simulink model "HEV_BTP_basic_Perfect_highway_final_25_11_19"  (R2019a)
settings: Solver=VariableStepAuto  StartTime=0  StopTime=198  RelTol=1e-3
undefined symbols (not defined in the file): f_co, f_co2, f_hc, f_nox, f_tbrake_n_bpt, f_tbrake_t_bpt, sigbuilder_block
libraries: fl_lib x100, nesl_utility x32, ee_lib x26, sdl_lib x17, simulink x5
(part 1 of 2)
settings Model: Creator=hp  LastModifiedBy=hp
settings SolverCC: ZeroCrossAlgorithm=Adaptive
settings DataIOCC: ExternalInput=[PedalTime,FrontBrakePedal,RearBrakePedal]  LoadExternalInput=on
settings DebuggingCC: IgnoredZcDiagnostic=none

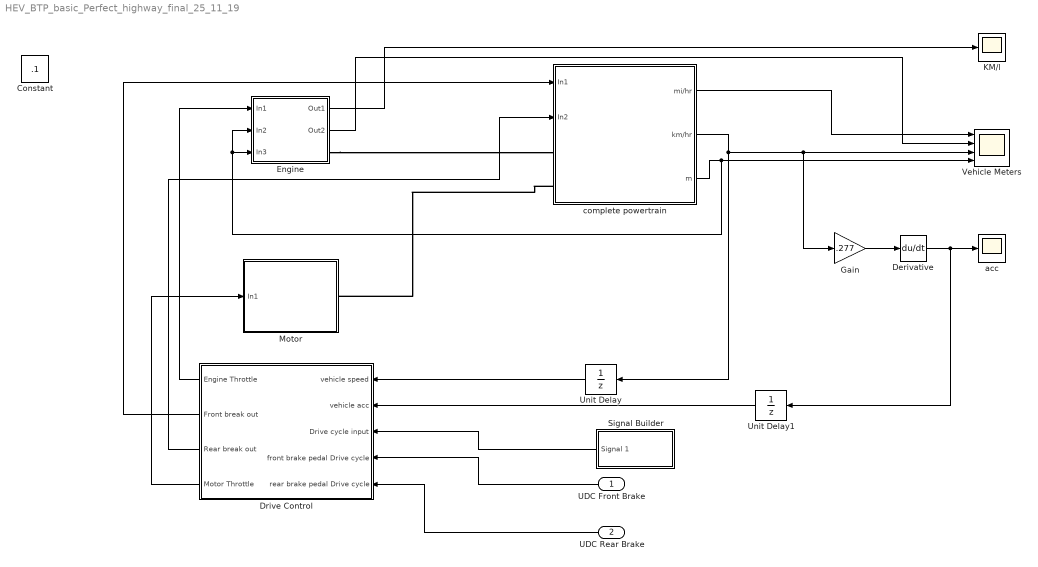
== system HEV_BTP_basic_Perfect_highway_final_25_11_19 ==
  UDC Front Brake : Inport
  UDC Rear Brake : Inport  Port=2
  Constant : Constant  Value=.1
  Derivative : Derivative
  Drive Control : Subsystem
  Engine : Subsystem
  Gain : Gain  Gain=.277
  KM/l : Scope
  Motor : Subsystem
  Signal Builder : Subsystem  Tag=STV Subsys  LoadFcn=sigbuilder_block('load');  StartFcn=sigbuilder_block('start');  StopFcn=sigbuilder_block('stop');  ClipboardFcn=sigbuilder_block('clipboard');  mask(Sigbuilder block){tuvar=[0:10]}
      mask help: Simulink:masks:SigbuilderBlock_MD
      mask init:
      | if ~strcmp(get_param(bdroot(gcbh),'SimulationStatus'),'stopped') tuvar = sigbuilder_block('maskInit'); end
      settings: CopyFcn=sigbuilder_block('copy');  DeleteFcn=sigbuilder_block('delete');  ModelCloseFcn=sigbuilder_block('modelClose');  PreSaveFcn=sigbuilder_block('preSave');  PauseFcn=sigbuilder_block('pause');  ContinueFcn=sigbuilder_block('continue');  NameChangeFcn=sigbuilder_block('namechange');  OpenFcn=sigbuilder_block('open',[6 30 1012.5 447.75 ]);  CloseFcn=sigbuilder_block('close');
      mask Display: plot(0, 0, 100, 100,[2, 2, 32, 32, 2], [68, 8, 8, 68, 68],[32, 2], [38, 38], [32, 19, 2],[53, 60, 44], [32, 17, 17, 2],[16, 16, 31, 31]);txt = getActiveGroup(gcbh);text(2, 100, txt,'verticalAlignment', 'top');
  Unit Delay : UnitDelay  SampleTime=-1  HasFrameUpgradeWarning=on
  Unit Delay1 : UnitDelay  SampleTime=-1  HasFrameUpgradeWarning=on
  "Vehicle Meters " : Scope  NumInputPorts=4
  acc : Scope
  complete powertrain : Subsystem
  wires:
  complete powertrain/2(km/hr) -> Unit Delay/1, Gain/1, "Vehicle Meters "/3
  complete powertrain/1(mi/hr) -> "Vehicle Meters "/1
  complete powertrain/3(m) -> Engine/2(In2), Engine/3(In3), "Vehicle Meters "/4
  Engine/1(Out1) -> KM/l/1
  Engine/2(Out2) -> "Vehicle Meters "/2
  Derivative/1 -> Unit Delay1/1, acc/1
  Gain/1 -> Derivative/1
  Drive Control/4(Motor Throttle) -> Motor/1(In1)
  Drive Control/1(Engine Throttle) -> Engine/1(In1)
  UDC Front Brake/1 -> Drive Control/4(front brake pedal Drive cycle)
  UDC Rear Brake/1 -> Drive Control/5(rear brake pedal Drive cycle)
  Drive Control/2(Front break out) -> complete powertrain/1(In1)
  Drive Control/3(Rear break out) -> complete powertrain/2(In2)
  Unit Delay/1 -> Drive Control/1(vehicle speed)
  Unit Delay1/1 -> Drive Control/2(vehicle acc)
  Signal Builder/1(Signal 1) -> Drive Control/3(Drive cycle input)
  connections:
  Engine/RConn1 -- complete powertrain/LConn1
  complete powertrain/LConn2 -- Motor/RConn1

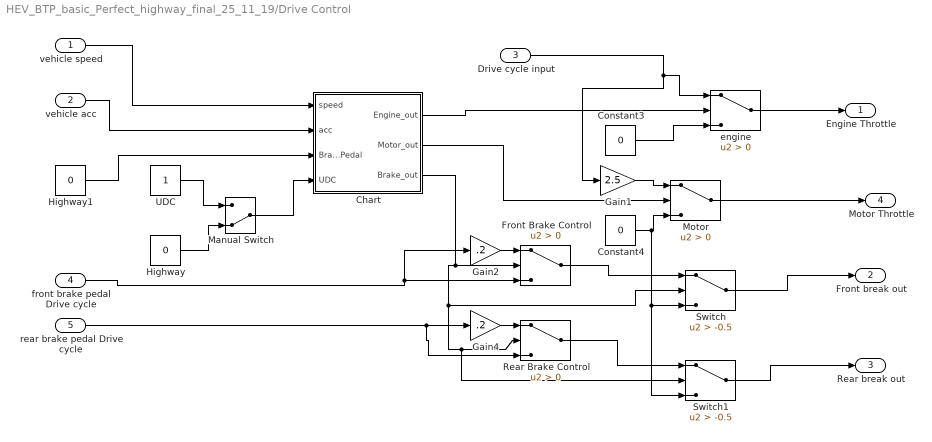
== system HEV_BTP_basic_Perfect_highway_final_25_11_19/Drive Control ==
  vehicle speed : Inport
  vehicle acc : Inport  Port=2
  Drive cycle input : Inport  Port=3
  front brake pedal Drive cycle : Inport  Port=4
  rear brake pedal Drive cycle : Inport  Port=5
  Chart : Stateflow chart  BlockKeywords=__PRM__SERIALIZED__DATA__:Stateflow Chart,Stateflow Diagram  TreatAsAtomicUnit=on
  Constant3 : Constant  Value=0
  Constant4 : Constant  Value=0
  Front Brake Control : Switch  Criteria=u2 > Threshold
  Gain1 : Gain  Gain=2.5
  Gain2 : Gain  Gain=.2
  Gain4 : Gain  Gain=.2
  Highway : Constant  Value=0
  Highway1 : Constant  Value=0
  Manual Switch : ManualSwitch  CurrentSetting=0
  Motor : Switch  Criteria=u2 > Threshold
  Rear Brake Control : Switch  Criteria=u2 > Threshold
  Switch : Switch  Criteria=u2 > Threshold  Threshold=-0.5
  Switch1 : Switch  Criteria=u2 > Threshold  Threshold=-0.5
  UDC : Constant
  engine : Switch  Criteria=u2 > Threshold
  Engine Throttle : Outport
  Front break out : Outport  Port=2
  Rear break out : Outport  Port=3
  Motor Throttle : Outport  Port=4
  wires:
  rear brake pedal Drive cycle/1 -> Rear Brake Control/3, Gain4/1
  Gain4/1 -> Rear Brake Control/1
  front brake pedal Drive cycle/1 -> Gain2/1, Front Brake Control/3
  Gain1/1 -> Motor/1
  Gain2/1 -> Front Brake Control/1
  UDC/1 -> Manual Switch/1
  Chart/2(Motor_out) -> Motor/2
  Chart/3(Brake_out) -> Front Brake Control/2, Switch/2, Switch1/2, Rear Brake Control/2
  Constant4/1 -> Switch1/3, Switch/3, Motor/3
  Highway/1 -> Manual Switch/2
  vehicle speed/1 -> Chart/1(speed)
  Drive cycle input/1 -> Gain1/1, engine/1
  engine/1 -> Engine Throttle/1
  Chart/1(Engine_out) -> engine/2
  Manual Switch/1 -> Chart/4(UDC)
  Constant3/1 -> engine/3
  Motor/1 -> Motor Throttle/1
  vehicle acc/1 -> Chart/2(acc)
  Front Brake Control/1 -> Switch/1
  Switch/1 -> Front break out/1
  Switch1/1 -> Rear break out/1
  Rear Brake Control/1 -> Switch1/1
  Highway1/1 -> Chart/3(Brake_Pedal)

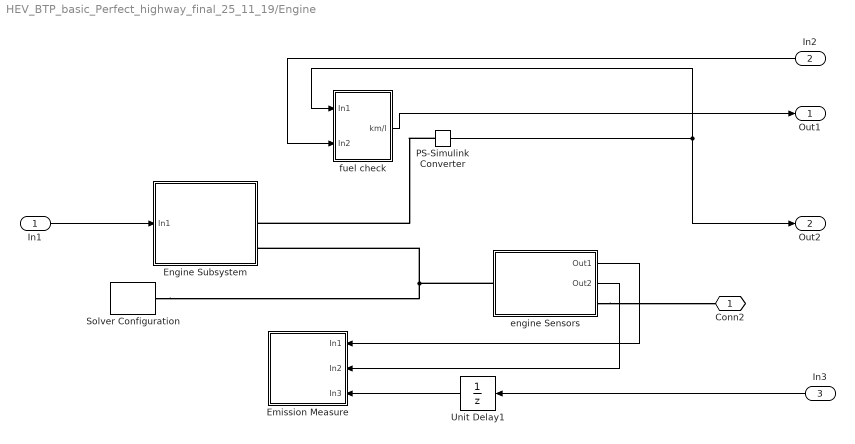
== system HEV_BTP_basic_Perfect_highway_final_25_11_19/Engine ==
  In1 : Inport
  In2 : Inport  Port=2
  In3 : Inport  Port=3
  Emission Measure : Subsystem
  Engine Subsystem : Subsystem
  PS-Simulink Converter : nesl_utility/PS-Simulink Converter  PhysicalDomain=network_engine_domain  SubClassName=ps_output  LeftPortType=input  RightPortType=output  PseudoPeriodic=off  Frequencies=[]  Unit=g/s  AffineConversion=off
  Solver Configuration : nesl_utility/Solver Configuration  PhysicalDomain=network_engine_domain  SubClassName=solver  LeftPortType=input  RightPortType=generic  Tones=[]  Harmonics=[]  SimulateNoise=off  Profile=off  UseLocalSampling=off  EnableSwitchedLinearOptims=on  FrequencyDomain=off  UseCCode=off  RelTol=0.001  AbsTol=1e-06  MinStep=1e-09  ToWorkspace=off  RevertToSquareIcSolve=off  NumHomotopyIterations=100  PhasorMode=off  PhasorModeNumHarmonics=1  DoDC=off  ResidualTolerance=1e-09  UseLocalSolver=off  LocalSolverChoice=NE_BACKWARD_EULER_ADVANCER  LocalSolverSampleTime=0.001  DoFixedCost=off  MaxNonlinIter=3  MaxModeIter=2  LinearAlgebra=auto  EquationFormulation=NE_TIME_EF  DelaysMemoryBudget=1024  AutomaticFiltering=on  FilteringTimeConstant=0.001  PartitionStorageMethod=AS_NEEDED  PartitionMemoryBudget=1024  PartitionMethod=ROBUST
  Unit Delay1 : UnitDelay  SampleTime=-1  HasFrameUpgradeWarning=on
  engine Sensors : Subsystem
  "fuel check " : Subsystem
  Conn2 : PMIOPort  Side=Right
  Out1 : Outport
  Out2 : Outport  Port=2
  wires:
  engine Sensors/1(Out1) -> Emission Measure/1(In1)
  Unit Delay1/1 -> Emission Measure/3(In3)
  "fuel check "/1(km/l) -> Out1/1
  engine Sensors/2(Out2) -> Emission Measure/2(In2)
  PS-Simulink Converter/1 -> Out2/1, "fuel check "/1(In1)
  In2/1 -> "fuel check "/2(In2)
  In3/1 -> Unit Delay1/1
  In1/1 -> Engine Subsystem/1(In1)
  connections:
  Solver Configuration/RConn1 -- engine Sensors/LConn1 -- Engine Subsystem/RConn3
  PS-Simulink Converter/LConn1 -- Engine Subsystem/RConn2
  engine Sensors/RConn1 -- Conn2/RConn1

== system HEV_BTP_basic_Perfect_highway_final_25_11_19/Motor ==
  In1 : Inport
  Battery Subsystem : Subsystem
  DC Motor : Subsystem
  Motor Sensors : Subsystem
  Conn1 : PMIOPort  Side=Right
  wires:
  In1/1 -> Battery Subsystem/1(Pedal Input)
  connections:
  Motor Sensors/LConn1 -- DC Motor/RConn1
  DC Motor/LConn1 -- Battery Subsystem/RConn1
  DC Motor/LConn2 -- Battery Subsystem/RConn2
  Motor Sensors/RConn1 -- Conn1/RConn1

== system HEV_BTP_basic_Perfect_highway_final_25_11_19/Signal Builder ==
  Demux : Demux  Tag=STV Demux  Outputs=1
  FromWs : FromWorkspace  Tag=STV FromWs  VariableName=tuvar  SampleTime=0
      SigBuilderData=|
      | common.afterFinalStr = 'Extrapolate'
      | common.sampleTime = 0
      | dataSet.timeRange = [0 200]
      | dataSet.name = 'Group 1'
      | sbobj.Groups.Name = 'Group 1'
      | sbobj.Groups.Signals.Name = 'Signal 1'
      | sbobj.Groups.Signals.XData = [0 3.33333333333 3.33333333333 6.66666666667 6.66666666667 12.6 14.8 16.6666666667 16.6666666667 20 23.3333333333 26.6666666667 30 33.3333333333 33.3333333333 36.6666666667 40 40 43.3333333333 46.6666666667 50 50 53.3333333333 56.6666666667 60 60 63.3333333333 63.3333333333 66.6666666667 66.6666666667 70 73.3333333333 76.6666666667 80 80 83.3333333333 86.6666666667 86.6666666667 90 90 93.3333333333 96.6666666667 96.6666666667 100 100 103.333333333 106.666666667 110 110 113.333333333 116.666666667 116.666666667 120 120 123.333333333 123.333333333 126.666666667 130 130 133.333333333 136.666666667 140 143.333333333 143.333333333 146.666666667 150 153.333333333 153.333333333 156.666666667 156.666666667 160 163.333333333 166.666666667 171 171 173.333333333 173.333333333 176.666666667 180 180 183.333333333 183.333333333 186.666666667 186.666666667 190 190 193.333333333 193.333333333 196.666666667 200]
      | sbobj.Groups.Signals.YData = [0.01 0.1 0.11 0.16 0.17 0.17 0.14 0.14 0.13 0.13 0.16 0.16 0.19 0.22 0.23 0.24 0.25 0.24 0.19 0.14 0.14 0.15 0.15 0.15 0.15 0.14 0.17 0.18 0.23 0.24 0.27 0.27 0.27 0.27 0.28 0.28 0.28 0.27 0.27 0.26 0.26 0.26 0.28 0.34 0.35 0.35 0.42 0.42 0.43 0.43 0.39 0.38 0.3 0.29 0.22 0.21 0.13 0.01 0 0 0 0.02 0.02 0.03 0.1 0.13 0.17 0.18 0.21 0.22 0.22 0.28 0.35 0.4 0.41 0.48 0.49 0.53 0.57 0.59 0.59 0.6 0.6 0.59 0.59 0.6 0.6 0.61 0.61 0.61]
      | sbobj.Groups.TimeRange = [0 200]
  Signal 1 : Outport  Tag=STV Outport
  wires:
  FromWs/1 -> Demux/1
  Demux/1 -> Signal 1/1

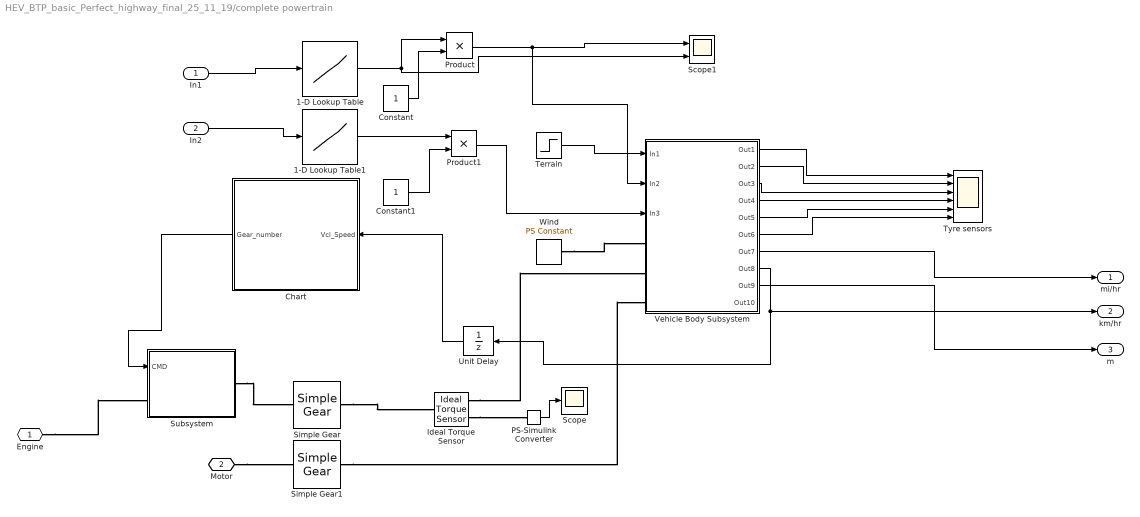
== system HEV_BTP_basic_Perfect_highway_final_25_11_19/complete powertrain ==
  In1 : Inport
  In2 : Inport  Port=2
  1-D Lookup Table : Lookup_n-D  NumberOfTableDimensions=1  BreakpointsForDimension1=0:0.01:1  Table=0:10:1000  InternalRulePriority=Speed  RndMeth=Simplest  InputSameDT=on
  1-D Lookup Table1 : Lookup_n-D  NumberOfTableDimensions=1  BreakpointsForDimension1=0:0.01:1  Table=0:10:1000  InternalRulePriority=Speed  RndMeth=Simplest  InputSameDT=on
  Chart : Stateflow chart  BlockKeywords=__PRM__SERIALIZED__DATA__:Stateflow Chart,Stateflow Diagram  TreatAsAtomicUnit=on
  Constant : Constant
  Constant1 : Constant
  Ideal Torque Sensor : fl_lib/Mechanical/Mechanical Sensors/Ideal Torque Sensor
  PS-Simulink Converter : nesl_utility/PS-Simulink Converter  PhysicalDomain=network_engine_domain  SubClassName=ps_output  LeftPortType=input  RightPortType=output  PseudoPeriodic=off  Frequencies=[]  Unit=N*m  AffineConversion=off
  Product : Product
  Product1 : Product
  Scope : Scope
  Scope1 : Scope  NumInputPorts=2
  Simple Gear : sdl_lib/Gears/Simple Gear  ratio=6  rotation_direction=1  friction_model=sdl.enum.gear_efficiencies_load.off  T_noload=0.1 N*m  T_nom=5 N*m  efficiency_nom=0.8  efficiency=0.8  mu_visc=[0, 0] N*m/(rad/s)  w_thr=0.01 rad/s  pwr_thr=0.001 W  enable_faults=simscape.enum.onoff.off  efficiency_fault=0.05  external_fault=simscape.enum.onoff.off  temporal_fault=simscape.enum.onoff.off  fault_time=5 s  fault_angles=pi / 12 rad  report_fault=1  temperature_TLU=[280, 300, 320] K  load_TLU=[1, 5, 10] N*m  efficiency_TLU=[.95, .9, .85]  efficiency_TLU2=[.85, .8, .75; .95, .9, .85; .85, .8, .7]  thermal_mass=50 J/K  T_init=300 K
      settings: SourceProductName=Simscape Driveline
  Simple Gear1 : sdl_lib/Gears/Simple Gear  ratio=12  rotation_direction=1  friction_model=sdl.enum.gear_efficiencies_load.off  T_noload=0.1 N*m  T_nom=5 N*m  efficiency_nom=0.8  efficiency=0.8  mu_visc=[0, 0] N*m/(rad/s)  w_thr=0.01 rad/s  pwr_thr=0.001 W  enable_faults=simscape.enum.onoff.off  efficiency_fault=0.05  external_fault=simscape.enum.onoff.off  temporal_fault=simscape.enum.onoff.off  fault_time=5 s  fault_angles=pi / 12 rad  report_fault=1  temperature_TLU=[280, 300, 320] K  load_TLU=[1, 5, 10] N*m  efficiency_TLU=[.95, .9, .85]  efficiency_TLU2=[.85, .8, .75; .95, .9, .85; .85, .8, .7]  thermal_mass=50 J/K  T_init=300 K
      settings: SourceProductName=Simscape Driveline
  Subsystem : Subsystem
  Terrain : Step  Time=700  Before=-0.5*(pi/180)  After=0  SampleTime=0
  Tyre sensors : Scope  NumInputPorts=6
  Unit Delay : UnitDelay  SampleTime=.05  HasFrameUpgradeWarning=on
  Vehicle Body Subsystem : Subsystem
  "Wind " : fl_lib/Physical Signals/Sources/PS Constant  constant=3 m/s
  Engine : PMIOPort  Side=Left
  Motor : PMIOPort  Port=2  Side=Left
  mi/hr : Outport
  km/hr : Outport  Port=2
  m : Outport  Port=3
  wires:
  Terrain/1 -> Vehicle Body Subsystem/1(In1)
  Vehicle Body Subsystem/1(Out1) -> Tyre sensors/1
  Vehicle Body Subsystem/3(Out3) -> Tyre sensors/3
  Vehicle Body Subsystem/6(Out6) -> Tyre sensors/6
  Vehicle Body Subsystem/5(Out5) -> Tyre sensors/5
  Vehicle Body Subsystem/2(Out2) -> Tyre sensors/2
  PS-Simulink Converter/1 -> Scope/1
  Vehicle Body Subsystem/4(Out4) -> Tyre sensors/4
  Chart/1(Gear_number) -> Subsystem/1("CMD ")
  Vehicle Body Subsystem/8(Out8) -> km/hr/1, Unit Delay/1
  Unit Delay/1 -> Chart/1(Vcl_Speed)
  Vehicle Body Subsystem/7(Out7) -> mi/hr/1
  Vehicle Body Subsystem/9(Out9) -> m/1
  In1/1 -> 1-D Lookup Table/1
  In2/1 -> 1-D Lookup Table1/1
  1-D Lookup Table/1 -> Product/1, Scope1/2
  Constant/1 -> Product/2
  Product/1 -> Vehicle Body Subsystem/2(In2), Scope1/1
  1-D Lookup Table1/1 -> Product1/1
  Constant1/1 -> Product1/2
  Product1/1 -> Vehicle Body Subsystem/3(In3)
  connections:
  Ideal Torque Sensor/RConn1 -- Vehicle Body Subsystem/LConn2
  "Wind "/RConn1 -- Vehicle Body Subsystem/LConn1
  Subsystem/RConn1 -- Simple Gear/LConn1
  Ideal Torque Sensor/RConn2 -- PS-Simulink Converter/LConn1
  Engine/RConn1 -- Subsystem/LConn1
  Simple Gear/RConn1 -- Ideal Torque Sensor/LConn1
  Simple Gear1/RConn1 -- Vehicle Body Subsystem/LConn3
  Motor/RConn1 -- Simple Gear1/LConn1

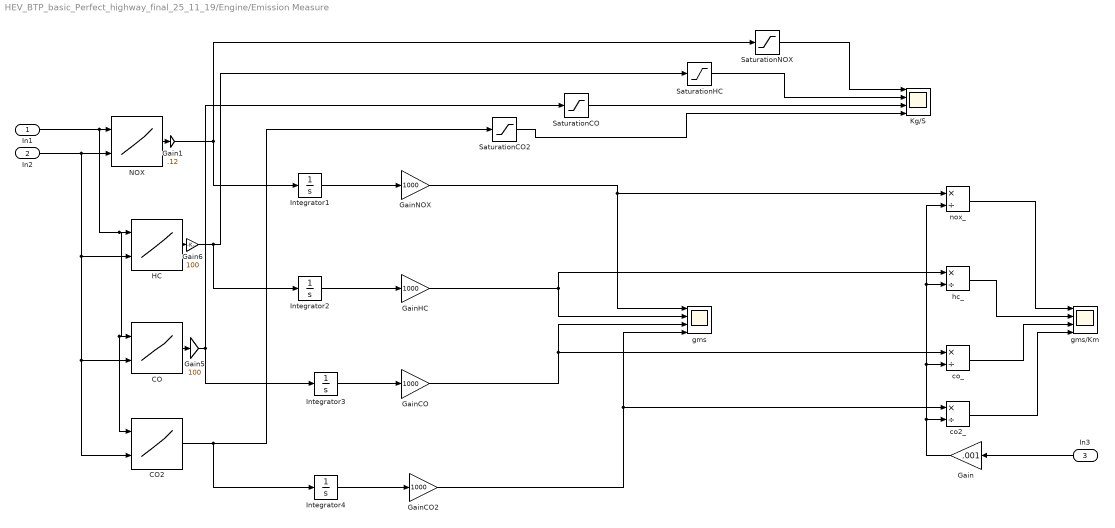
== system HEV_BTP_basic_Perfect_highway_final_25_11_19/Engine/Emission Measure ==
  In1 : Inport
  In2 : Inport  Port=2
  In3 : Inport  Port=3
  CO : Lookup_n-D  BreakpointsForDimension1=f_tbrake_t_bpt  BreakpointsForDimension2=f_tbrake_n_bpt  Table=f_co  InternalRulePriority=Speed  RndMeth=Simplest  InputSameDT=on
  CO2 : Lookup_n-D  BreakpointsForDimension1=f_tbrake_t_bpt  BreakpointsForDimension2=f_tbrake_n_bpt  Table=f_co2  InternalRulePriority=Speed  RndMeth=Simplest  InputSameDT=on
  Gain : Gain  Gain=.001
  Gain1 : Gain  Gain=.12
  Gain5 : Gain  Gain=100
  Gain6 : Gain  Gain=100
  GainCO : Gain  Gain=1000
  GainCO2 : Gain  Gain=1000
  GainHC : Gain  Gain=1000
  GainNOX : Gain  Gain=1000
  HC : Lookup_n-D  BreakpointsForDimension1=f_tbrake_t_bpt  BreakpointsForDimension2=f_tbrake_n_bpt  Table=f_hc  InternalRulePriority=Speed  RndMeth=Simplest  InputSameDT=on
  Integrator{1..4} (4 alike) : Integrator
  Kg/S : Scope  NumInputPorts=4
  NOX : Lookup_n-D  BreakpointsForDimension1=f_tbrake_t_bpt  BreakpointsForDimension2=f_tbrake_n_bpt  Table=f_nox  InternalRulePriority=Speed  RndMeth=Simplest  InputSameDT=on
  SaturationCO : Saturate  UpperLimit=inf  LowerLimit=0  ZeroCross=off
  SaturationCO2 : Saturate  UpperLimit=inf  LowerLimit=0  ZeroCross=off
  SaturationHC : Saturate  UpperLimit=inf  LowerLimit=0  ZeroCross=off
  SaturationNOX : Saturate  UpperLimit=inf  LowerLimit=0  ZeroCross=off
  co2_ : Product  Inputs=*/
  co_ : Product  Inputs=*/
  gms : Scope  NumInputPorts=4
  gms/Km : Scope  NumInputPorts=4
  hc_ : Product  Inputs=*/
  nox_ : Product  Inputs=*/
  wires:
  NOX/1 -> Gain1/1
  In2/1 -> CO2/2, CO/2, HC/2, NOX/2
  In1/1 -> CO2/1, CO/1, HC/1, NOX/1
  HC/1 -> Gain6/1
  CO/1 -> Gain5/1
  CO2/1 -> SaturationCO2/1, Integrator4/1
  SaturationNOX/1 -> Kg/S/1
  SaturationHC/1 -> Kg/S/2
  SaturationCO2/1 -> Kg/S/4
  SaturationCO/1 -> Kg/S/3
  Gain6/1 -> Integrator2/1, SaturationHC/1
  Gain5/1 -> SaturationCO/1, Integrator3/1
  Integrator3/1 -> GainCO/1
  Integrator4/1 -> GainCO2/1
  Integrator2/1 -> GainHC/1
  Integrator1/1 -> GainNOX/1
  GainCO2/1 -> co2_/1, gms/4
  GainHC/1 -> gms/2, hc_/1
  GainNOX/1 -> nox_/1, gms/1
  GainCO/1 -> gms/3, co_/1
  Gain/1 -> nox_/2, hc_/2, co_/2, co2_/2
  nox_/1 -> gms/Km/1
  hc_/1 -> gms/Km/2
  co_/1 -> gms/Km/3
  co2_/1 -> gms/Km/4
  Gain1/1 -> SaturationNOX/1, Integrator1/1
  In3/1 -> Gain/1

== system HEV_BTP_basic_Perfect_highway_final_25_11_19/Engine/Engine Subsystem ==
  In1 : Inport
  Generic Engine : sdl_lib/Engines/Generic Engine  model_parameterization=1  engine_type=1  P_max=51.5 kW  w_P_max=5500 rpm  w_max=6175 rpm  w_min=500 rpm  w_tab=[500, 1000, 2000, 3000, 4000, 5000, 6000, 7000] rpm  trq_tab=[380, 380, 380, 380, 350, 280, 200, 80] N*m  pwr_tab=[20, 40, 78, 120, 145, 148, 125, 60] kW  interp_method=simscape.enum.interpolation.linear  model_inertia=1  inertia=.5 kg*m^2  initial_velocity=875 rpm  model_time_constant=0  time_constant=0.2 s  T0=0  w_thr=100 rpm  idle_speed=0  idle_speed_reference=1000 rpm  tau_controller=1 s  idle_w_thr=1 rpm  redline=0  redline_speed=5000 rpm  tau_redline=1 s  redline_w_thr=1 rpm  fc_model=2  fc_per_rev=22.816 mg/rev  displaced_volume=400 cm^3  rev_per_cycle=2  fc_w_tab=[875, 2000, 3000, 4000, 5000, 6175] rpm  fc_trq_tab=[0, 80, 160, 200, 240, 320, 360, 400] N*m  fc_tab=[0.75, 0.45, 0.7, 0.8, 0.95, 1.35, 1.7, 2.2; 0.5, 0.85, 1.35, 1.55, 1.8, 2.5, 3, 3.7; 0.7, 1.35, 2, 2.4, 2.8, 3.75, 4.25, 5.25; 1, 1.8, 2.9, 3.35, 4, 5.35, 5.85, 6.65; 1.25, 2.4, 3.95, 4.7, 5.4, 7, 8.1, 9.3; 1.55, 3, 5.15, 5.95, 6.9, 9.2, 11, 13.25] g/s  bmep_tab=[0, 250, 500, 625, 750, 1000, 1150, 1250] kPa  bsfc_tab=[410, 380, 300, 280, 270, 290, 320, 380; 410, 370, 290, 270, 260, 270, 285, 320; 415, 380, 290, 275, 265, 270, 270, 300; 420, 390, 310, 290, 285, 280, 280, 285; 430, 410, 340, 320, 310, 300, 310, 320; 450, 430, 370, 340, 330, 330, 350, 380] g/hr/kW  fc_interp_method=simscape.enum.interpolation.linear
      settings: SourceProductName=Simscape Driveline  SourceProductBaseCode=LD  LogSimulationData=on
  Mechanical Rotational Reference : fl_lib/Mechanical/Rotational Elements/Mechanical Rotational Reference
  Simulink-PS Converter : nesl_utility/Simulink-PS Converter  PhysicalDomain=network_engine_domain  SubClassName=ps_input  LeftPortType=input  RightPortType=output  PseudoPeriodic=off  Frequencies=[]  NoiseDistribution=none  NoiseParameters=[]  Unit=1  AffineConversion=off  FilteringAndDerivatives=provide  SimscapeFilterOrder=1  InputFilterTimeConstant=0.001  UdotUserProvided=0
  Conn1 : PMIOPort  Side=Right
  Conn2 : PMIOPort  Port=2  Side=Right
  Conn3 : PMIOPort  Port=3  Side=Right
  wires:
  In1/1 -> Simulink-PS Converter/1
  connections:
  Simulink-PS Converter/RConn1 -- Generic Engine/LConn1
  Generic Engine/RConn1 -- Conn1/RConn1
  Mechanical Rotational Reference/LConn1 -- Generic Engine/LConn2
  Conn3/RConn1 -- Generic Engine/RConn3
  Generic Engine/RConn2 -- Conn2/RConn1

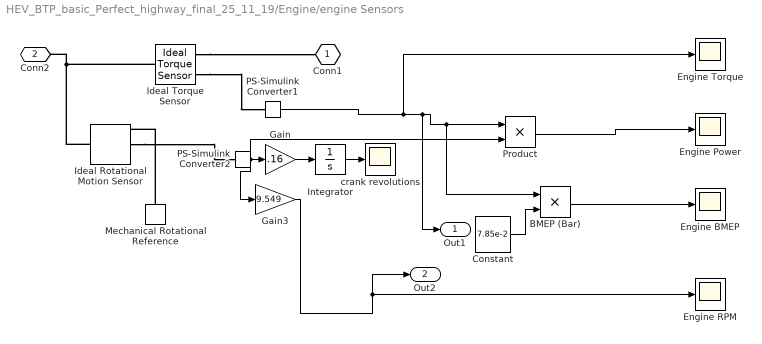
== system HEV_BTP_basic_Perfect_highway_final_25_11_19/Engine/engine Sensors ==
  BMEP (Bar) : Product
  Constant : Constant  Value=7.85e-2
  Engine BMEP : Scope
  Engine Power : Scope
  Engine Torque : Scope
  Engine RPM : Scope
  Gain : Gain  Gain=.16
  Gain3 : Gain  Gain=9.549
  Ideal Rotational Motion Sensor : fl_lib/Mechanical/Mechanical Sensors/Ideal Rotational Motion Sensor  offset=0 rad
  Ideal Torque Sensor : fl_lib/Mechanical/Mechanical Sensors/Ideal Torque Sensor
  Integrator : Integrator
  Mechanical Rotational Reference : fl_lib/Mechanical/Rotational Elements/Mechanical Rotational Reference
  PS-Simulink Converter1 : nesl_utility/PS-Simulink Converter  PhysicalDomain=network_engine_domain  SubClassName=ps_output  LeftPortType=input  RightPortType=output  PseudoPeriodic=off  Frequencies=[]  Unit=N*m  AffineConversion=off
  PS-Simulink Converter2 : nesl_utility/PS-Simulink Converter  PhysicalDomain=network_engine_domain  SubClassName=ps_output  LeftPortType=input  RightPortType=output  PseudoPeriodic=off  Frequencies=[]  Unit=rad/s  AffineConversion=off
  Product : Product
  crank revolutions : Scope
  Conn1 : PMIOPort  Side=Right
  Conn2 : PMIOPort  Port=2  Side=Left
  Out1 : Outport
  Out2 : Outport  Port=2
  wires:
  PS-Simulink Converter2/1 -> Product/2, Gain3/1, Gain/1
  Product/1 -> Engine Power/1
  PS-Simulink Converter1/1 -> Out1/1, BMEP (Bar)/1, Product/1, Engine Torque/1
  Gain/1 -> Integrator/1
  Integrator/1 -> crank revolutions/1
  Gain3/1 -> Out2/1, Engine RPM/1
  Constant/1 -> BMEP (Bar)/2
  BMEP (Bar)/1 -> Engine BMEP/1
  connections:
  Ideal Rotational Motion Sensor/LConn1 -- Conn2/RConn1 -- Ideal Torque Sensor/LConn1
  Mechanical Rotational Reference/LConn1 -- Ideal Rotational Motion Sensor/RConn1
  Ideal Torque Sensor/RConn2 -- PS-Simulink Converter1/LConn1
  Ideal Torque Sensor/RConn1 -- Conn1/RConn1
  Ideal Rotational Motion Sensor/RConn2 -- PS-Simulink Converter2/LConn1

== system HEV_BTP_basic_Perfect_highway_final_25_11_19/Engine/fuel check  ==
  In1 : Inport
  In2 : Inport  Port=2
  Divide : Product  Inputs=*/
  Integrator : Integrator
  fuel grams : Scope
  to km : Gain  Gain=1/1000
  to liters : Gain  Gain=1/770
  km/l : Outport
  wires:
  Integrator/1 -> to liters/1, fuel grams/1
  In2/1 -> to km/1
  to liters/1 -> Divide/2
  Divide/1 -> km/l/1
  In1/1 -> Integrator/1
  to km/1 -> Divide/1

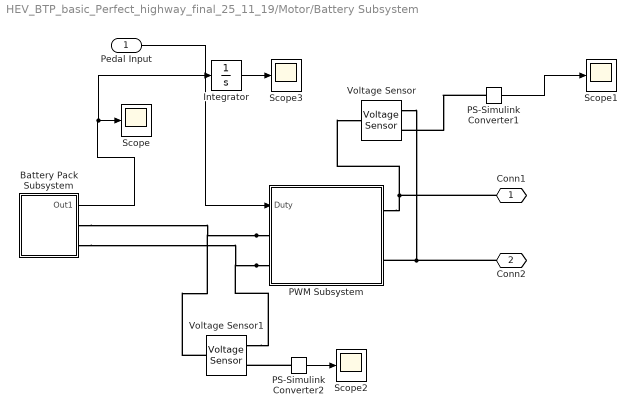
== system HEV_BTP_basic_Perfect_highway_final_25_11_19/Motor/Battery Subsystem ==
  Pedal Input : Inport
  Battery Pack Subsystem : Subsystem
  Integrator : Integrator
  PS-Simulink Converter1 : nesl_utility/PS-Simulink Converter  PhysicalDomain=network_engine_domain  SubClassName=ps_output  LeftPortType=input  RightPortType=output  PseudoPeriodic=off  Frequencies=[]  Unit=V  AffineConversion=off
  PS-Simulink Converter2 : nesl_utility/PS-Simulink Converter  PhysicalDomain=network_engine_domain  SubClassName=ps_output  LeftPortType=input  RightPortType=output  PseudoPeriodic=off  Frequencies=[]  Unit=V  AffineConversion=off
  PWM Subsystem : Subsystem
  Scope{,1..3} (4 alike) : Scope
  Voltage Sensor : fl_lib/Electrical/Electrical Sensors/Voltage Sensor
  Voltage Sensor1 : fl_lib/Electrical/Electrical Sensors/Voltage Sensor
  Conn1 : PMIOPort  Side=Right
  Conn2 : PMIOPort  Port=2  Side=Right
  wires:
  PS-Simulink Converter1/1 -> Scope1/1
  Pedal Input/1 -> PWM Subsystem/1(Duty)
  PS-Simulink Converter2/1 -> Scope2/1
  Battery Pack Subsystem/1(Out1) -> Integrator/1, Scope/1
  Integrator/1 -> Scope3/1
  connections:
  PWM Subsystem/LConn2 -- Battery Pack Subsystem/RConn2 -- Voltage Sensor1/RConn2
  PWM Subsystem/LConn1 -- Battery Pack Subsystem/RConn1 -- Voltage Sensor1/LConn1
  PS-Simulink Converter1/LConn1 -- Voltage Sensor/RConn1
  Voltage Sensor/RConn2 -- PWM Subsystem/RConn2 -- Conn2/RConn1
  PS-Simulink Converter2/LConn1 -- Voltage Sensor1/RConn1
  Conn1/RConn1 -- PWM Subsystem/RConn1 -- Voltage Sensor/LConn1

== system HEV_BTP_basic_Perfect_highway_final_25_11_19/Motor/DC Motor ==
  DC Motor : ee_lib/Electromechanical/Brushed Motors/DC Motor  parameterization=1  Ra=0.0093 Ohm  La=172 uH  emf_or_torque=2  Kv=0.19 V/(rad/s)  Ki=0.19 N*m/A  T_stall=2.4e-4 N*m  w_max=15000 rpm  w_rated=10000 rpm  P_rated=10 kW  V_rated=48 V  J=0.001 kg*m^2  lam_param=1  lam=1e-6 N*m/(rad/s)  i_noload=0 A  V_i_noload=1.5 V  speed0=0 rad/s  alpha=3.93e-3 1/K  Tmeas=25 degC  thermal_mass=100 J/K  initial_temperature=25 degC
      settings: SourceProductName=Simscape Electrical
  Electrical Reference2 : fl_lib/Electrical/Electrical Elements/Electrical Reference
  Mechanical Rotational Reference : fl_lib/Mechanical/Rotational Elements/Mechanical Rotational Reference
  Conn1 : PMIOPort  Side=Left
  Conn2 : PMIOPort  Port=2  Side=Right
  Conn3 : PMIOPort  Port=3  Side=Left
  connections:
  DC Motor/LConn1 -- Conn1/RConn1
  DC Motor/RConn2 -- Mechanical Rotational Reference/LConn1
  DC Motor/LConn2 -- Conn2/RConn1
  Electrical Reference2/LConn1 -- DC Motor/RConn1 -- Conn3/RConn1

== system HEV_BTP_basic_Perfect_highway_final_25_11_19/Motor/Motor Sensors ==
  Gain : Gain  Gain=9.549
  Ideal Rotational Motion Sensor : fl_lib/Mechanical/Mechanical Sensors/Ideal Rotational Motion Sensor  offset=0 rad
  Ideal Torque Sensor : fl_lib/Mechanical/Mechanical Sensors/Ideal Torque Sensor
  Mechanical Rotational Reference1 : fl_lib/Mechanical/Rotational Elements/Mechanical Rotational Reference
  Motor Power : Scope
  Motor RPM : Scope
  Motor Torque : Scope
  PS-Simulink Converter : nesl_utility/PS-Simulink Converter  PhysicalDomain=network_engine_domain  SubClassName=ps_output  LeftPortType=input  RightPortType=output  PseudoPeriodic=off  Frequencies=[]  Unit=N*m  AffineConversion=off
  PS-Simulink Converter3 : nesl_utility/PS-Simulink Converter  PhysicalDomain=network_engine_domain  SubClassName=ps_output  LeftPortType=input  RightPortType=output  PseudoPeriodic=off  Frequencies=[]  Unit=rad/s  AffineConversion=off
  Product : Product
  Conn1 : PMIOPort  Side=Right
  Conn2 : PMIOPort  Port=2  Side=Left
  wires:
  PS-Simulink Converter3/1 -> Product/2, Gain/1
  Product/1 -> Motor Power/1
  PS-Simulink Converter/1 -> Product/1, Motor Torque/1
  Gain/1 -> Motor RPM/1
  connections:
  Ideal Torque Sensor/LConn1 -- Ideal Rotational Motion Sensor/LConn1 -- Conn2/RConn1
  Ideal Torque Sensor/RConn2 -- PS-Simulink Converter/LConn1
  PS-Simulink Converter3/LConn1 -- Ideal Rotational Motion Sensor/RConn2
  Mechanical Rotational Reference1/LConn1 -- Ideal Rotational Motion Sensor/RConn1
  Ideal Torque Sensor/RConn1 -- Conn1/RConn1

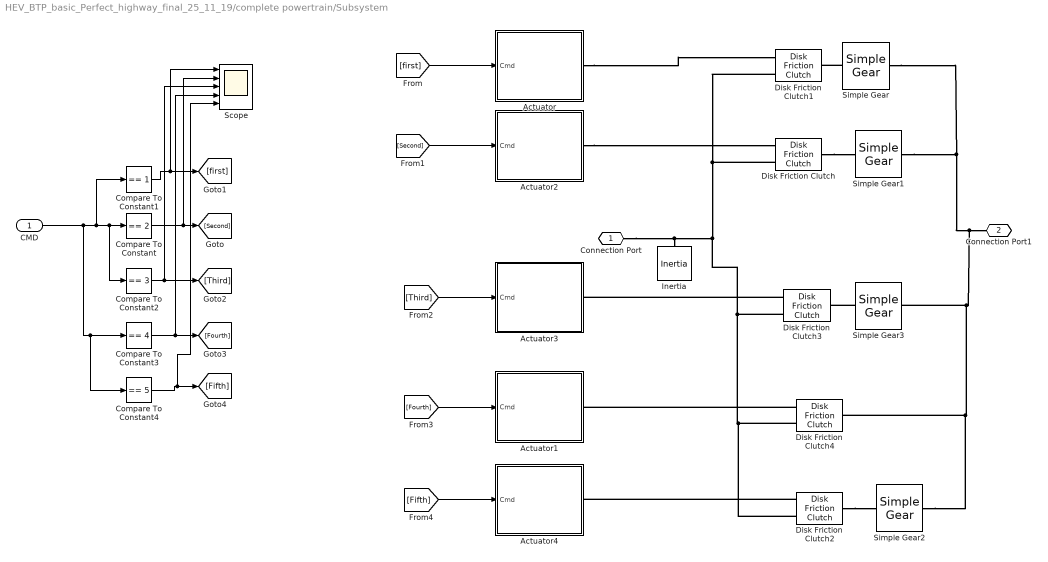
== system HEV_BTP_basic_Perfect_highway_final_25_11_19/complete powertrain/Subsystem ==
  "CMD " : Inport
  Actuator : Subsystem
  Actuator1 : Subsystem
  Actuator2 : Subsystem
  Actuator3 : Subsystem
  Actuator4 : Subsystem
  Compare To Constant : simulink/Logic and Bit Operations/Compare To Constant  relop===  const=2  OutDataTypeStr=boolean
  Compare To Constant1 : simulink/Logic and Bit Operations/Compare To Constant  relop===  const=1  OutDataTypeStr=boolean
  Compare To Constant2 : simulink/Logic and Bit Operations/Compare To Constant  relop===  const=3  OutDataTypeStr=boolean
  Compare To Constant3 : simulink/Logic and Bit Operations/Compare To Constant  relop===  const=4  OutDataTypeStr=boolean
  Compare To Constant4 : simulink/Logic and Bit Operations/Compare To Constant  relop===  const=5  OutDataTypeStr=boolean
  Disk Friction Clutch{,1..4} (5 alike) : sdl_lib/Clutches/Disk Friction Clutch  geometry_model=1  r_eff=130 mm  d_o=150 mm  d_i=100 mm  nS=4  piston_area=0.001 m^2  unidirectional=0  friction_model=1  mu_coulomb=0.3  mu_w_vector=[0, 100, 1000] rad/s  mu_coulomb_vector=[.3, .22, .19]  mu_interp_method=simscape.enum.interpolation.linear  mu_extrap_method=simscape.enum.extrapolation.linear  mu_static=0.35  d_f=1  w_tol=0.001 rad/s  pressure_min=100 Pa  mu_visc=0 N*m/(rad/s)  initial_state_locked=0  temperature_TLU=[280, 300, 320] K  mu_coulomb_temp_vector=[.3, .28, .25]  mu_coulomb_matrix=[.34, .32, .3; .3, .28, .25; .25, .2, .15]  mu_static_vector=[.4, .38, .36]  thermal_mass=25 kJ/K  T_init=300 K
      settings: SourceProductName=Simscape Driveline  SourceProductBaseCode=LD
  Inertia : fl_lib/Mechanical/Rotational Elements/Inertia  inertia=0.01 kg*m^2  w_specify=on  w_priority=None  w=0 rad/s  w_nominal_specify=off  w_nominal_unit=rad/s  w_nominal_value=1  t_specify=off  t_priority=None  t=0 N*m  t_nominal_specify=off  t_nominal_unit=N*m  t_nominal_value=1
  Scope : Scope  NumInputPorts=5
  Simple Gear : sdl_lib/Gears/Simple Gear  ratio=2.95  rotation_direction=1  friction_model=sdl.enum.gear_efficiencies_load.off  T_noload=0.1 N*m  T_nom=5 N*m  efficiency_nom=0.8  efficiency=0.8  mu_visc=[0, 0] N*m/(rad/s)  w_thr=0.01 rad/s  pwr_thr=0.001 W  enable_faults=simscape.enum.onoff.off  efficiency_fault=0.05  external_fault=simscape.enum.onoff.off  temporal_fault=simscape.enum.onoff.off  fault_time=5 s  fault_angles=pi / 12 rad  report_fault=1  temperature_TLU=[280, 300, 320] K  load_TLU=[1, 5, 10] N*m  efficiency_TLU=[.95, .9, .85]  efficiency_TLU2=[.85, .8, .75; .95, .9, .85; .85, .8, .7]  thermal_mass=50 J/K  T_init=300 K
      settings: SourceProductName=Simscape Driveline
  Simple Gear1 : sdl_lib/Gears/Simple Gear  ratio=1.94  rotation_direction=1  friction_model=sdl.enum.gear_efficiencies_load.off  T_noload=0.1 N*m  T_nom=5 N*m  efficiency_nom=0.8  efficiency=0.8  mu_visc=[0, 0] N*m/(rad/s)  w_thr=0.01 rad/s  pwr_thr=0.001 W  enable_faults=simscape.enum.onoff.off  efficiency_fault=0.05  external_fault=simscape.enum.onoff.off  temporal_fault=simscape.enum.onoff.off  fault_time=5 s  fault_angles=pi / 12 rad  report_fault=1  temperature_TLU=[280, 300, 320] K  load_TLU=[1, 5, 10] N*m  efficiency_TLU=[.95, .9, .85]  efficiency_TLU2=[.85, .8, .75; .95, .9, .85; .85, .8, .7]  thermal_mass=50 J/K  T_init=300 K
      settings: SourceProductName=Simscape Driveline
  Simple Gear2 : sdl_lib/Gears/Simple Gear  ratio=.68  rotation_direction=1  friction_model=sdl.enum.gear_efficiencies_load.off  T_noload=0.1 N*m  T_nom=5 N*m  efficiency_nom=0.8  efficiency=0.8  mu_visc=[0, 0] N*m/(rad/s)  w_thr=0.01 rad/s  pwr_thr=0.001 W  enable_faults=simscape.enum.onoff.off  efficiency_fault=0.05  external_fault=simscape.enum.onoff.off  temporal_fault=simscape.enum.onoff.off  fault_time=5 s  fault_angles=pi / 12 rad  report_fault=1  temperature_TLU=[280, 300, 320] K  load_TLU=[1, 5, 10] N*m  efficiency_TLU=[.95, .9, .85]  efficiency_TLU2=[.85, .8, .75; .95, .9, .85; .85, .8, .7]  thermal_mass=50 J/K  T_init=300 K
      settings: SourceProductName=Simscape Driveline
  Simple Gear3 : sdl_lib/Gears/Simple Gear  ratio=1.34  rotation_direction=1  friction_model=sdl.enum.gear_efficiencies_load.off  T_noload=0.1 N*m  T_nom=5 N*m  efficiency_nom=0.8  efficiency=0.8  mu_visc=[0, 0] N*m/(rad/s)  w_thr=0.01 rad/s  pwr_thr=0.001 W  enable_faults=simscape.enum.onoff.off  efficiency_fault=0.05  external_fault=simscape.enum.onoff.off  temporal_fault=simscape.enum.onoff.off  fault_time=5 s  fault_angles=pi / 12 rad  report_fault=1  temperature_TLU=[280, 300, 320] K  load_TLU=[1, 5, 10] N*m  efficiency_TLU=[.95, .9, .85]  efficiency_TLU2=[.85, .8, .75; .95, .9, .85; .85, .8, .7]  thermal_mass=50 J/K  T_init=300 K
      settings: SourceProductName=Simscape Driveline
  Connection Port : PMIOPort  Side=Left
  Connection Port1 : PMIOPort  Port=2  Side=Right
  wires:
  Compare To Constant/1 -> Scope/2, [Second]
  [first] -> Actuator/1(Cmd)
  Compare To Constant1/1 -> Scope/1, [first]
  Compare To Constant2/1 -> Scope/3, [Third]
  Compare To Constant3/1 -> Scope/4, [Fourth]
  "CMD "/1 -> Compare To Constant2/1, Compare To Constant/1, Compare To Constant1/1, Compare To Constant4/1, Compare To Constant3/1
  [Second] -> Actuator2/1(Cmd)
  [Third] -> Actuator3/1(Cmd)
  [Fourth] -> Actuator1/1(Cmd)
  Compare To Constant4/1 -> Scope/5, [Fifth]
  [Fifth] -> Actuator4/1(Cmd)
  connections:
  Disk Friction Clutch/RConn1 -- Simple Gear1/LConn1
  Disk Friction Clutch/LConn2 -- Inertia/LConn1 -- Connection Port/RConn1 -- Disk Friction Clutch2/LConn2 -- Disk Friction Clutch4/LConn2 -- Disk Friction Clutch3/LConn2 -- Disk Friction Clutch1/LConn2
  Actuator/RConn1 -- Disk Friction Clutch1/LConn1
  Actuator2/RConn1 -- Disk Friction Clutch/LConn1
  Disk Friction Clutch3/LConn1 -- Actuator3/RConn1
  Disk Friction Clutch4/LConn1 -- Actuator1/RConn1
  Simple Gear/LConn1 -- Disk Friction Clutch1/RConn1
  Simple Gear1/RConn1 -- Simple Gear/RConn1 -- Disk Friction Clutch4/RConn1 -- Simple Gear2/RConn1 -- Simple Gear3/RConn1 -- Connection Port1/RConn1
  Disk Friction Clutch2/RConn1 -- Simple Gear2/LConn1
  Disk Friction Clutch2/LConn1 -- Actuator4/RConn1
  Simple Gear3/LConn1 -- Disk Friction Clutch3/RConn1

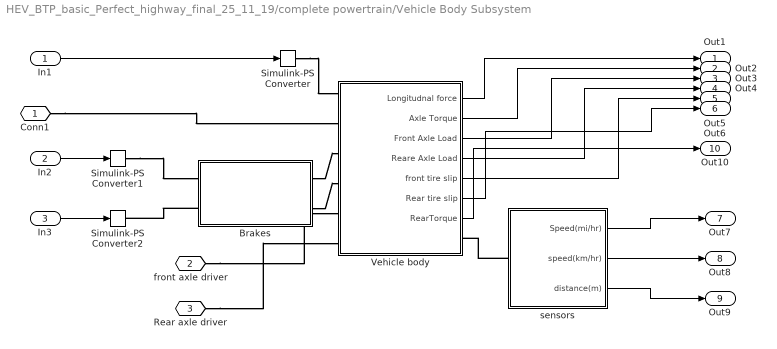
== system HEV_BTP_basic_Perfect_highway_final_25_11_19/complete powertrain/Vehicle Body Subsystem ==
  In1 : Inport
  In2 : Inport  Port=2
  In3 : Inport  Port=3
  Brakes : Subsystem
  Simulink-PS Converter : nesl_utility/Simulink-PS Converter  PhysicalDomain=network_engine_domain  SubClassName=ps_input  LeftPortType=input  RightPortType=output  PseudoPeriodic=off  Frequencies=[]  NoiseDistribution=none  NoiseParameters=[]  Unit=1  AffineConversion=off  FilteringAndDerivatives=provide  SimscapeFilterOrder=1  InputFilterTimeConstant=0.001  UdotUserProvided=0
  Simulink-PS Converter1 : nesl_utility/Simulink-PS Converter  PhysicalDomain=network_engine_domain  SubClassName=ps_input  LeftPortType=input  RightPortType=output  PseudoPeriodic=off  Frequencies=[]  NoiseDistribution=none  NoiseParameters=[]  Unit=N  AffineConversion=off  FilteringAndDerivatives=provide  SimscapeFilterOrder=1  InputFilterTimeConstant=0.001  UdotUserProvided=0
  Simulink-PS Converter2 : nesl_utility/Simulink-PS Converter  PhysicalDomain=network_engine_domain  SubClassName=ps_input  LeftPortType=input  RightPortType=output  PseudoPeriodic=off  Frequencies=[]  NoiseDistribution=none  NoiseParameters=[]  Unit=N  AffineConversion=off  FilteringAndDerivatives=provide  SimscapeFilterOrder=1  InputFilterTimeConstant=0.001  UdotUserProvided=0
  Vehicle body : Subsystem
  sensors : Subsystem
  Conn1 : PMIOPort  Side=Left
  front axle driver : PMIOPort  Port=2  Side=Left
  Rear axle driver : PMIOPort  Port=3  Side=Left
  Out1 : Outport
  Out2 : Outport  Port=2
  Out3 : Outport  Port=3
  Out4 : Outport  Port=4
  Out5 : Outport  Port=5
  Out6 : Outport  Port=6
  Out7 : Outport  Port=7
  Out8 : Outport  Port=8
  Out9 : Outport  Port=9
  Out10 : Outport  Port=10
  wires:
  Vehicle body/1(Longitudnal force) -> Out1/1
  Vehicle body/2(Axle Torque) -> Out2/1
  sensors/1(Speed(mi/hr)) -> Out7/1
  Vehicle body/5(front tire slip) -> Out5/1
  Vehicle body/6(Rear tire slip) -> Out6/1
  sensors/2(speed(km/hr)) -> Out8/1
  In1/1 -> Simulink-PS Converter/1
  In3/1 -> Simulink-PS Converter2/1
  sensors/3("distance(m) ") -> Out9/1
  In2/1 -> Simulink-PS Converter1/1
  Vehicle body/3(Front Axle Load) -> Out3/1
  Vehicle body/4(Reare Axle Load) -> Out4/1
  Vehicle body/7(RearTorque) -> Out10/1
  connections:
  Simulink-PS Converter1/RConn1 -- Brakes/LConn1
  Brakes/LConn2 -- Simulink-PS Converter2/RConn1
  sensors/LConn1 -- Vehicle body/RConn1
  Brakes/RConn1 -- Vehicle body/LConn3
  Brakes/RConn2 -- Vehicle body/LConn4
  Simulink-PS Converter/RConn1 -- Vehicle body/LConn1
  Conn1/RConn1 -- Vehicle body/LConn2
  front axle driver/RConn1 -- Vehicle body/LConn5
  Rear axle driver/RConn1 -- Vehicle body/LConn6

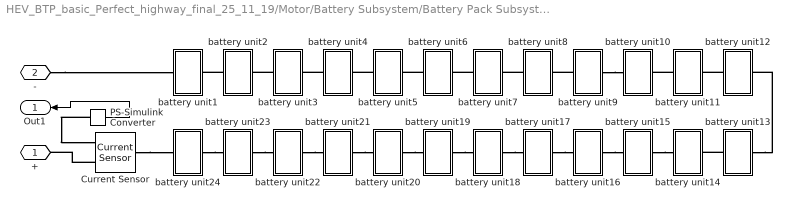
== system HEV_BTP_basic_Perfect_highway_final_25_11_19/Motor/Battery Subsystem/Battery Pack Subsystem ==
  Current Sensor : fl_lib/Electrical/Electrical Sensors/Current Sensor
  PS-Simulink Converter : nesl_utility/PS-Simulink Converter  PhysicalDomain=network_engine_domain  SubClassName=ps_output  LeftPortType=input  RightPortType=output  PseudoPeriodic=off  Frequencies=[]  Unit=A  AffineConversion=off
  battery unit1 : Subsystem
  battery unit10 : Subsystem
  battery unit11 : Subsystem
  battery unit12 : Subsystem
  battery unit13 : Subsystem
  battery unit14 : Subsystem
  battery unit15 : Subsystem
  battery unit16 : Subsystem
  battery unit17 : Subsystem
  battery unit18 : Subsystem
  battery unit19 : Subsystem
  battery unit2 : Subsystem
  battery unit20 : Subsystem
  battery unit21 : Subsystem
  battery unit22 : Subsystem
  battery unit23 : Subsystem
  battery unit24 : Subsystem
  battery unit3 : Subsystem
  battery unit4 : Subsystem
  battery unit5 : Subsystem
  battery unit6 : Subsystem
  battery unit7 : Subsystem
  battery unit8 : Subsystem
  battery unit9 : Subsystem
  + : PMIOPort  Side=Right
  - : PMIOPort  Port=2  Side=Right
  Out1 : Outport
  wires:
  PS-Simulink Converter/1 -> Out1/1
  connections:
  battery unit24/LConn1 -- battery unit23/RConn1
  battery unit5/LConn1 -- battery unit4/RConn1
  battery unit17/LConn1 -- battery unit16/RConn1
  battery unit20/LConn1 -- battery unit19/RConn1
  battery unit3/LConn1 -- battery unit2/RConn1
  battery unit22/LConn1 -- battery unit21/RConn1
  battery unit8/LConn1 -- battery unit7/RConn1
  battery unit6/LConn1 -- battery unit5/RConn1
  battery unit2/LConn1 -- battery unit1/RConn1
  battery unit16/LConn1 -- battery unit15/RConn1
  battery unit18/LConn1 -- battery unit17/RConn1
  battery unit7/LConn1 -- battery unit6/RConn1
  battery unit19/LConn1 -- battery unit18/RConn1
  battery unit11/LConn1 -- battery unit10/RConn1
  battery unit13/LConn1 -- battery unit12/RConn1
  battery unit15/LConn1 -- battery unit14/RConn1
  battery unit21/LConn1 -- battery unit20/RConn1
  battery unit9/RConn1 -- battery unit10/LConn1
  battery unit23/LConn1 -- battery unit22/RConn1
  battery unit12/LConn1 -- battery unit11/RConn1
  battery unit4/LConn1 -- battery unit3/RConn1
  battery unit9/LConn1 -- battery unit8/RConn1
  battery unit13/RConn1 -- battery unit14/LConn1
  PS-Simulink Converter/LConn1 -- Current Sensor/RConn1
  -/RConn1 -- battery unit1/LConn1
  Current Sensor/RConn2 -- +/RConn1
  Current Sensor/LConn1 -- battery unit24/RConn1

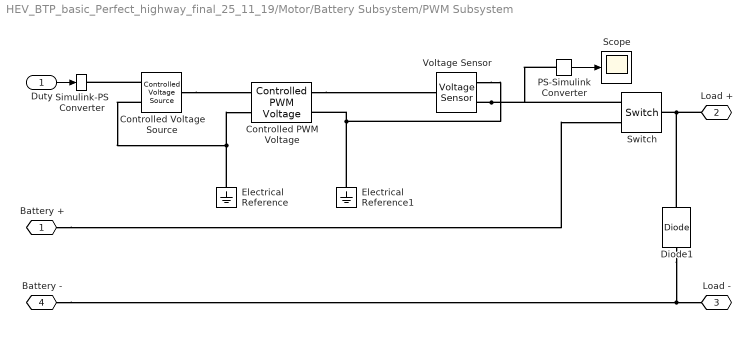
== system HEV_BTP_basic_Perfect_highway_final_25_11_19/Motor/Battery Subsystem/PWM Subsystem ==
  Duty : Inport
  Controlled PWM Voltage : ee_lib/Integrated Circuits/Controlled PWM Voltage  F=.1 kHz  TD=0 s  pulse_width_offset=0 s  pulse_min=0 s  Vmin=0 V  Vmax=1 V  Vm=48 V  pwm_or_av=1  event_type=1  sample_time=1e-6 s  u_min=0  u_max=1
      settings: SourceProductName=Simscape Electrical
  Controlled Voltage Source : fl_lib/Electrical/Electrical Sources/Controlled Voltage Source
  Diode1 : fl_lib/Electrical/Electrical Elements/Diode  Vf=0.6 V  Ron=0.3 Ohm  Goff=1e-8 1/Ohm  i_specify=off  i_priority=None  i=0 A  i_nominal_specify=off  i_nominal_unit=A  i_nominal_value=1  v_specify=off  v_priority=None  v=0 V  v_nominal_specify=off  v_nominal_unit=V  v_nominal_value=1
  Electrical Reference : fl_lib/Electrical/Electrical Elements/Electrical Reference
  Electrical Reference1 : fl_lib/Electrical/Electrical Elements/Electrical Reference
  PS-Simulink Converter : nesl_utility/PS-Simulink Converter  PhysicalDomain=network_engine_domain  SubClassName=ps_output  LeftPortType=input  RightPortType=output  PseudoPeriodic=off  Frequencies=[]  Unit=1  AffineConversion=off
  Scope : Scope
  Simulink-PS Converter : nesl_utility/Simulink-PS Converter  PhysicalDomain=network_engine_domain  SubClassName=ps_input  LeftPortType=input  RightPortType=output  PseudoPeriodic=off  Frequencies=[]  NoiseDistribution=none  NoiseParameters=[]  Unit=1  AffineConversion=off  FilteringAndDerivatives=provide  SimscapeFilterOrder=1  InputFilterTimeConstant=0.001  UdotUserProvided=0
  Switch : fl_lib/Electrical/Electrical Elements/Switch  R_closed=0.01 Ohm  G_open=1e-8 1/Ohm  Threshold=0  i_specify=off  i_priority=None  i=0 A  i_nominal_specify=off  i_nominal_unit=A  i_nominal_value=1  v_specify=off  v_priority=None  v=0 V  v_nominal_specify=off  v_nominal_unit=V  v_nominal_value=1
      settings: SourceProductName=Simscape
  Voltage Sensor : fl_lib/Electrical/Electrical Sensors/Voltage Sensor
  Battery + : PMIOPort  Side=Left
  Load + : PMIOPort  Port=2  Side=Right
  Load - : PMIOPort  Port=3  Side=Right
  Battery - : PMIOPort  Port=4  Side=Left
  wires:
  Duty/1 -> Simulink-PS Converter/1
  PS-Simulink Converter/1 -> Scope/1
  connections:
  Controlled Voltage Source/RConn1 -- Simulink-PS Converter/RConn1
  Controlled PWM Voltage/RConn1 -- Voltage Sensor/LConn1
  Voltage Sensor/RConn1 -- Switch/RConn1 -- PS-Simulink Converter/LConn1
  Electrical Reference1/LConn1 -- Controlled PWM Voltage/RConn2 -- Voltage Sensor/RConn2
  Electrical Reference/LConn1 -- Controlled Voltage Source/RConn2 -- Controlled PWM Voltage/LConn2
  Controlled Voltage Source/LConn1 -- Controlled PWM Voltage/LConn1
  Battery +/RConn1 -- Switch/RConn2
  Load +/RConn1 -- Diode1/RConn1 -- Switch/LConn1
  Battery -/RConn1 -- Diode1/LConn1 -- Load -/RConn1

== system HEV_BTP_basic_Perfect_highway_final_25_11_19/complete powertrain/Subsystem/Actuator ==
  Cmd : Inport
  P<Pth : Constant  Value=0
  P>Pth : Constant  Value=1e7
  Simulink-PS Converter : nesl_utility/Simulink-PS Converter  PhysicalDomain=network_engine_domain  SubClassName=ps_input  LeftPortType=input  RightPortType=output  PseudoPeriodic=off  Frequencies=[]  NoiseDistribution=none  NoiseParameters=[]  Unit=1  AffineConversion=off  FilteringAndDerivatives=provide  SimscapeFilterOrder=1  InputFilterTimeConstant=0.001  UdotUserProvided=0
  Switch : Switch  Criteria=u2 > Threshold  Threshold=0.5
  Presure : PMIOPort  Side=Right
  wires:
  Cmd/1 -> Switch/2
  Switch/1 -> Simulink-PS Converter/1
  P<Pth/1 -> Switch/3
  P>Pth/1 -> Switch/1
  connections:
  Simulink-PS Converter/RConn1 -- Presure/RConn1

== system HEV_BTP_basic_Perfect_highway_final_25_11_19/complete powertrain/Subsystem/Actuator1 ==
  Cmd : Inport
  P<Pth : Constant  Value=0
  P>Pth : Constant  Value=1e7
  Simulink-PS Converter : nesl_utility/Simulink-PS Converter  PhysicalDomain=network_engine_domain  SubClassName=ps_input  LeftPortType=input  RightPortType=output  PseudoPeriodic=off  Frequencies=[]  NoiseDistribution=none  NoiseParameters=[]  Unit=1  AffineConversion=off  FilteringAndDerivatives=provide  SimscapeFilterOrder=1  InputFilterTimeConstant=0.001  UdotUserProvided=0
  Switch : Switch  Criteria=u2 > Threshold  Threshold=0.5
  Presure : PMIOPort  Side=Right
  wires:
  P>Pth/1 -> Switch/1
  P<Pth/1 -> Switch/3
  Switch/1 -> Simulink-PS Converter/1
  Cmd/1 -> Switch/2
  connections:
  Simulink-PS Converter/RConn1 -- Presure/RConn1

== system HEV_BTP_basic_Perfect_highway_final_25_11_19/complete powertrain/Subsystem/Actuator2 ==
  Cmd : Inport
  P<Pth : Constant  Value=0
  P>Pth : Constant  Value=1e7
  Simulink-PS Converter : nesl_utility/Simulink-PS Converter  PhysicalDomain=network_engine_domain  SubClassName=ps_input  LeftPortType=input  RightPortType=output  PseudoPeriodic=off  Frequencies=[]  NoiseDistribution=none  NoiseParameters=[]  Unit=1  AffineConversion=off  FilteringAndDerivatives=provide  SimscapeFilterOrder=1  InputFilterTimeConstant=0.001  UdotUserProvided=0
  Switch : Switch  Criteria=u2 > Threshold  Threshold=.5
  Presure : PMIOPort  Side=Right
  wires:
  P>Pth/1 -> Switch/1
  P<Pth/1 -> Switch/3
  Switch/1 -> Simulink-PS Converter/1
  Cmd/1 -> Switch/2
  connections:
  Simulink-PS Converter/RConn1 -- Presure/RConn1

== system HEV_BTP_basic_Perfect_highway_final_25_11_19/complete powertrain/Subsystem/Actuator3 ==
  Cmd : Inport
  P<Pth : Constant  Value=0
  P>Pth : Constant  Value=1e7
  Simulink-PS Converter : nesl_utility/Simulink-PS Converter  PhysicalDomain=network_engine_domain  SubClassName=ps_input  LeftPortType=input  RightPortType=output  PseudoPeriodic=off  Frequencies=[]  NoiseDistribution=none  NoiseParameters=[]  Unit=1  AffineConversion=off  FilteringAndDerivatives=provide  SimscapeFilterOrder=1  InputFilterTimeConstant=0.001  UdotUserProvided=0
  Switch : Switch  Criteria=u2 > Threshold  Threshold=0.5
  Presure : PMIOPort  Side=Right
  wires:
  P>Pth/1 -> Switch/1
  P<Pth/1 -> Switch/3
  Switch/1 -> Simulink-PS Converter/1
  Cmd/1 -> Switch/2
  connections:
  Simulink-PS Converter/RConn1 -- Presure/RConn1

== system HEV_BTP_basic_Perfect_highway_final_25_11_19/complete powertrain/Subsystem/Actuator4 ==
  Cmd : Inport
  P<Pth : Constant  Value=0
  P>Pth : Constant  Value=1e7
  Simulink-PS Converter : nesl_utility/Simulink-PS Converter  PhysicalDomain=network_engine_domain  SubClassName=ps_input  LeftPortType=input  RightPortType=output  PseudoPeriodic=off  Frequencies=[]  NoiseDistribution=none  NoiseParameters=[]  Unit=1  AffineConversion=off  FilteringAndDerivatives=provide  SimscapeFilterOrder=1  InputFilterTimeConstant=0.001  UdotUserProvided=0
  Switch : Switch  Criteria=u2 > Threshold  Threshold=0.5
  Presure : PMIOPort  Side=Right
  wires:
  Cmd/1 -> Switch/2
  Switch/1 -> Simulink-PS Converter/1
  P<Pth/1 -> Switch/3
  P>Pth/1 -> Switch/1
  connections:
  Simulink-PS Converter/RConn1 -- Presure/RConn1

== system HEV_BTP_basic_Perfect_highway_final_25_11_19/complete powertrain/Vehicle Body Subsystem/Brakes ==
  Loaded-Contact Rotational Friction : sdl_lib/Brakes & Detents/Rotational/Loaded-Contact Rotational Friction  geometry_model=1  r_eff=130 mm  d_o=150 mm  d_i=100 mm  friction_model=1  mu_coulomb=0.3  mu_w_vector=[0, 100, 1000] rad/s  mu_coulomb_vector=[.3, .22, .19]  mu_interp_method=simscape.enum.interpolation.linear  mu_extrap_method=simscape.enum.extrapolation.linear  mu_static=0.35  w_tol=0.001 rad/s  force_min=10 N  mu_visc=0 N*m/(rad/s)  initial_state_locked=0  temperature_TLU=[280, 300, 320] K  mu_coulomb_temp_vector=[.3, .28, .25]  mu_coulomb_matrix=[.34, .32, .3; .3, .28, .25; .25, .2, .15]  mu_static_vector=[.4, .38, .36]  thermal_mass=50 kJ/K  T_init=300 K
      settings: SourceProductName=Simscape Driveline  SourceProductBaseCode=LD
  Loaded-Contact Rotational Friction1 : sdl_lib/Brakes & Detents/Rotational/Loaded-Contact Rotational Friction  geometry_model=1  r_eff=130 mm  d_o=150 mm  d_i=100 mm  friction_model=1  mu_coulomb=0.3  mu_w_vector=[0, 100, 1000] rad/s  mu_coulomb_vector=[.3, .22, .19]  mu_interp_method=simscape.enum.interpolation.linear  mu_extrap_method=simscape.enum.extrapolation.linear  mu_static=0.35  w_tol=0.001 rad/s  force_min=10 N  mu_visc=0 N*m/(rad/s)  initial_state_locked=0  temperature_TLU=[280, 300, 320] K  mu_coulomb_temp_vector=[.3, .28, .25]  mu_coulomb_matrix=[.34, .32, .3; .3, .28, .25; .25, .2, .15]  mu_static_vector=[.4, .38, .36]  thermal_mass=50 kJ/K  T_init=300 K
      settings: SourceProductName=Simscape Driveline  SourceProductBaseCode=LD
  Mechanical Rotational Reference : fl_lib/Mechanical/Rotational Elements/Mechanical Rotational Reference
  Mechanical Rotational Reference1 : fl_lib/Mechanical/Rotational Elements/Mechanical Rotational Reference
  Front brake force : PMIOPort  Side=Left
  fB : PMIOPort  Port=2  Side=Right
  Rear brake force : PMIOPort  Port=3  Side=Left
  rB : PMIOPort  Port=4  Side=Right
  connections:
  Mechanical Rotational Reference1/LConn1 -- Loaded-Contact Rotational Friction1/LConn2
  Loaded-Contact Rotational Friction/RConn1 -- fB/RConn1
  Mechanical Rotational Reference/LConn1 -- Loaded-Contact Rotational Friction/LConn2
  Loaded-Contact Rotational Friction/LConn1 -- Front brake force/RConn1
  Loaded-Contact Rotational Friction1/RConn1 -- rB/RConn1
  Loaded-Contact Rotational Friction1/LConn1 -- Rear brake force/RConn1

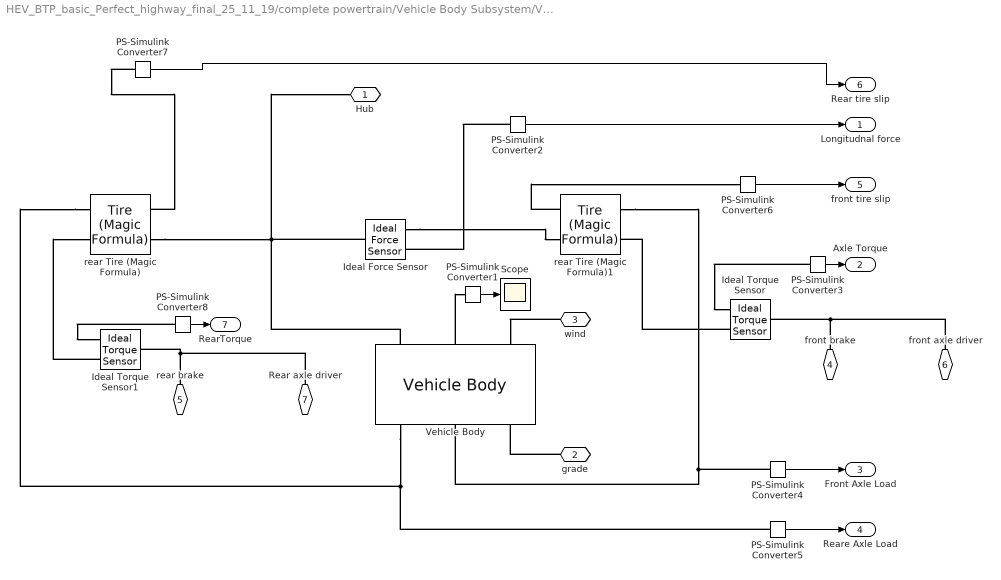
== system HEV_BTP_basic_Perfect_highway_final_25_11_19/complete powertrain/Vehicle Body Subsystem/Vehicle body ==
  Ideal Force Sensor : fl_lib/Mechanical/Mechanical Sensors/Ideal Force Sensor
  Ideal Torque Sensor : fl_lib/Mechanical/Mechanical Sensors/Ideal Torque Sensor
  Ideal Torque Sensor1 : fl_lib/Mechanical/Mechanical Sensors/Ideal Torque Sensor
  PS-Simulink Converter{1..8} (8 alike) : nesl_utility/PS-Simulink Converter  PhysicalDomain=network_engine_domain  SubClassName=ps_output  LeftPortType=input  RightPortType=output  PseudoPeriodic=off  Frequencies=[]  Unit=1  AffineConversion=off
  Scope : Scope
  Vehicle Body : sdl_lib/Tires & Vehicles/Vehicle Body  mass=1200 kg  n_w=1  x_f=1.160 m  x_r=1.325 m  y_c=0.5 m  mass_var=simscape.enum.onoff.off  model_pitch=simscape.enum.onoff.off  inertia=4000 kg*m^2  suspension_model=sdl.enum.linearTLU.linear  k_f=1e4 N/m  b_f=1e4 N/(m/s)  k_r=1e4 N/m  b_r=1e4 N/(m/s)  k_f_TLU=[-2000, -1000, 0, 1000, 2000] N  x_f_TLU=[-.4, -.2, 0, .2, .4] m  b_f_TLU=[-200, -100, 0, 100, 200] N  v_f_TLU=[-4, -2, 0, 2, 4] m/s  k_r_TLU=[-2000, -1000, 0, 1000, 2000] N  x_r_TLU=[-.4, -.2, 0, .2, .4] m  b_r_TLU=[-200, -100, 0, 100, 200] N  v_r_TLU=[-4, -2, 0, 2, 4] m/s  interp_method=simscape.enum.interpolation.linear  extrap_method=simscape.enum.extrapolation.linear  model_hardstop=simscape.enum.onoff.off  upper_bound_f=.25 m  lower_bound_f=-.25 m  stop_k_f=1e6 N/m  stop_b_f=150 N/(m/s)  upper_bound_r=.25 m  lower_bound_r=-.25 m  stop_k_r=1e6 N/m  stop_b_r=150 N/(m/s)  initial_pitch=0 rad  initial_pitch_rate=0 rad/s  g=9.81 m/s^2  liftoff_warning=simscape.enum.onoff.off  area=1.78 m^2  Cd=0.3  rho=1.225 kg/m^3  v_specify=off  v_priority=High  v=0 m/s  v_nominal_specify=off  v_nominal_unit=m/s  v_nominal_value=1
      settings: SourceProductName=Simscape Driveline
  rear Tire (Magic Formula) : sdl_lib/Tires & Vehicles/Tire (Magic Formula)  parameterization=sdl.enum.magic_tire_model.constant  F_z1=3000 N  F_x1=3500 N  kappa1=10  B_m=10  C_m=1.9  D_m=1  E_m=0.97  fz0=4000 N  p_Cx=1.685  p_Dx=[1.21, -.037]  p_Ex=[.344, .095, -.02, 0]  p_Kx=[21.51, -.163, .245]  p_Hx=[-.002, .002]  p_Vx=[0, 0]  v_tr_thr=0.1 m/s  r_e=.27 m  model_compliance=0  stiffness=1e6 N/m  damping=1000 N/(m/s)  model_inertia=1  inertia=.51 kg*m^2  initial_velocity=0 rad/s  model_resistance=1  resistance_model=1  coeff=0.015  p_tire=250e3 Pa  alpha=-0.003  beta=0.97  coeff_a=84e-4  coeff_b=6.2e-4 s/m  coeff_c=1.6e-4 s^2/m^2  v_thr=0.001 m/s
      settings: SourceProductName=Simscape Driveline
  rear Tire (Magic Formula)1 : sdl_lib/Tires & Vehicles/Tire (Magic Formula)  parameterization=sdl.enum.magic_tire_model.constant  F_z1=3000 N  F_x1=3500 N  kappa1=10  B_m=10  C_m=1.9  D_m=1  E_m=0.97  fz0=4000 N  p_Cx=1.685  p_Dx=[1.21, -.037]  p_Ex=[.344, .095, -.02, 0]  p_Kx=[21.51, -.163, .245]  p_Hx=[-.002, .002]  p_Vx=[0, 0]  v_tr_thr=0.1 m/s  r_e=.27 m  model_compliance=0  stiffness=1e6 N/m  damping=1000 N/(m/s)  model_inertia=1  inertia=.51 kg*m^2  initial_velocity=0 rad/s  model_resistance=1  resistance_model=1  coeff=0.015  p_tire=250e3 Pa  alpha=-0.003  beta=0.97  coeff_a=84e-4  coeff_b=6.2e-4 s/m  coeff_c=1.6e-4 s^2/m^2  v_thr=0.001 m/s
      settings: SourceProductName=Simscape Driveline
  Hub : PMIOPort  Side=Right
  grade : PMIOPort  Port=2  Side=Left
  wind : PMIOPort  Port=3  Side=Left
  front brake : PMIOPort  Port=4  Side=Left
  rear brake : PMIOPort  Port=5  Side=Left
  front axle driver : PMIOPort  Port=6  Side=Left
  Rear axle driver : PMIOPort  Port=7  Side=Left
  Longitudnal force : Outport
  Axle Torque : Outport  Port=2
  Front Axle Load : Outport  Port=3
  Reare Axle Load : Outport  Port=4
  front tire slip : Outport  Port=5
  Rear tire slip : Outport  Port=6
  RearTorque : Outport  Port=7
  wires:
  PS-Simulink Converter1/1 -> Scope/1
  PS-Simulink Converter2/1 -> Longitudnal force/1
  PS-Simulink Converter3/1 -> Axle Torque/1
  PS-Simulink Converter4/1 -> Front Axle Load/1
  PS-Simulink Converter5/1 -> Reare Axle Load/1
  PS-Simulink Converter6/1 -> front tire slip/1
  PS-Simulink Converter7/1 -> Rear tire slip/1
  PS-Simulink Converter8/1 -> RearTorque/1
  connections:
  Vehicle Body/LConn2 -- PS-Simulink Converter1/LConn1
  Ideal Torque Sensor/RConn1 -- rear Tire (Magic Formula)1/LConn2
  rear Tire (Magic Formula)/LConn1 -- Vehicle Body/RConn1 -- PS-Simulink Converter5/LConn1
  PS-Simulink Converter7/LConn1 -- rear Tire (Magic Formula)/RConn1
  rear Tire (Magic Formula)1/LConn1 -- Vehicle Body/RConn2 -- PS-Simulink Converter4/LConn1
  wind/RConn1 -- Vehicle Body/LConn3
  rear Tire (Magic Formula)/RConn2 -- Hub/RConn1 -- Ideal Force Sensor/LConn1 -- Vehicle Body/LConn1
  rear Tire (Magic Formula)1/RConn1 -- PS-Simulink Converter6/LConn1
  grade/RConn1 -- Vehicle Body/RConn3
  Ideal Force Sensor/RConn1 -- rear Tire (Magic Formula)1/RConn2
  PS-Simulink Converter2/LConn1 -- Ideal Force Sensor/RConn2
  PS-Simulink Converter3/LConn1 -- Ideal Torque Sensor/RConn2
  front axle driver/RConn1 -- front brake/RConn1 -- Ideal Torque Sensor/LConn1
  Ideal Torque Sensor1/RConn1 -- rear Tire (Magic Formula)/LConn2
  PS-Simulink Converter8/LConn1 -- Ideal Torque Sensor1/RConn2
  rear brake/RConn1 -- Rear axle driver/RConn1 -- Ideal Torque Sensor1/LConn1
